simulink model "IndustrialMicrogrid"  (R2025a)
settings: Solver=FixedStepAuto  StartTime=0.0  StopTime=8  FixedStep=Ts  RelTol=1e-3
PostLoadFcn:
  | IndustrialMicrogridInputData
  | GfmGridFormingConverterInputParameters
model workspace (MAT data in the model file):
  caseNum = 2
undefined symbols (not defined in the file): base, BESS, DiscIntNeverNeededParam, grid, Grid, gridInverter, machine, microgrid, PV, PVInverter, PVTransformer, scrFactorRg, scrFactorXg, transformer, Transition_and_Dispatch_ControlModeType, Ts
libraries: ee_lib x126, fl_lib x91, eeGeneralControl x73, nesl_utility x50, nesl_utility_internal x46, simulink x30, eeTransforms x11, eeSinusoidalMeasurementV2 x5, eeTotalHarmonicDistorsion x4, slpidlib x3, simulink_extras x2, eePowerMeasurement x2
(part 5 of 12)

== system IndustrialMicrogrid/MG2 Processing, Lighting and Auxiliary Loads/Motor Loads ==
  Asynchronous Machine Squirrel Cage (fundamental) : ee_lib/Electromechanical/Asynchronous/Induction Machine Squirrel Cage  port_option=ee.enum.threePhasePort.composite  SRated=750000 V*A  VRated=4160 V  FRated=60 Hz  nPolePairs=2  param_unit=ee.enum.unit.si  squirrel_cage=ee.enum.squirrelcage.Single  zero_sequence=ee.enum.park.zerosequence.exclude  initialization_option=ee.enum.asm.initialization.fluxvariables  Rs=0.016744*7 Ohm  Xls=0.035490*7 Ohm  pu_Rs=0.0258  pu_Lls=0.0413  Rrd=0.009857*7 Ohm  Xlrd=0.04280*7 Ohm  pu_Rrd=0.0145  pu_Llrd=0.0424  Rrd1=0.28 Ohm  Xlrd1=0.82 Ohm  Rrd2=0.28 Ohm  Xlrd2=0.82 Ohm  pu_Rrd1=0.0290  pu_Llrd1=0.0848  pu_Rrd2=0.0290  pu_Llrd2=0.0848  Xm=111.90*7 Ohm  pu_Lm=1.7562  X0=0.4*7 Ohm  pu_L0=0.0413  saturation_option=ee.enum.saturation.exclude  saturation_i=[0, 4, 9, 18, 25, 34, 50, 68, 95, 120] A  saturation_v=[0, 88, 154, 198, 220, 242, 264, 286, 308, 327] V  pu_saturation_i=[0, .176, .396, .792, 1.1, 1.496, 2.2, 2.992, 4.18, 5.28]  pu_saturation_v=[0, .4, .7, .9, 1, 1.1, 1.2, 1.3, 1.4, 1.4864]  connection_option=ee.enum.Connection.delta1  angular_position_specify=off  angular_position_priority=None  angular_position=0 deg  angular_position_nominal_specify=off  angular_position_nominal_value=1  angular_position_nominal_unit=deg  pu_psids_specify=off  pu_psids_priority=None  pu_psids=0  pu_psids_nominal_specify=off  pu_psids_nominal_value=1  pu_psids_nominal_unit=1  pu_psiqs_specify=off  pu_psiqs_priority=None  pu_psiqs=0  pu_psiqs_nominal_specify=off  pu_psiqs_nominal_value=1  pu_psiqs_nominal_unit=1  pu_psi0s_specify=off  pu_psi0s_priority=None  pu_psi0s=0  pu_psi0s_nominal_specify=off  pu_psi0s_nominal_value=1  pu_psi0s_nominal_unit=1  pu_psidr_specify=off  pu_psidr_priority=None  pu_psidr=0  pu_psidr_nominal_specify=off  pu_psidr_nominal_value=1  pu_psidr_nominal_unit=1  pu_psiqr_specify=off  pu_psiqr_priority=None  pu_psiqr=0  pu_psiqr_nominal_specify=off  pu_psiqr_nominal_value=1  pu_psiqr_nominal_unit=1  pu_psidr1_specify=off  pu_psidr1_priority=None  pu_psidr1=0  pu_psidr1_nominal_specify=off  pu_psidr1_nominal_value=1  pu_psidr1_nominal_unit=1  pu_psiqr1_specify=off  pu_psiqr1_priority=None  pu_psiqr1=0  pu_psiqr1_nominal_specify=off  pu_psiqr1_nominal_value=1  pu_psiqr1_nominal_unit=1  pu_psidr2_specify=off  pu_psidr2_priority=None  pu_psidr2=0  pu_psidr2_nominal_specify=off  pu_psidr2_nominal_value=1  pu_psidr2_nominal_unit=1  pu_psiqr2_specify=off  pu_psiqr2_priority=None  pu_psiqr2=0  pu_psiqr2_nominal_specify=off  pu_psiqr2_nominal_value=1  pu_psiqr2_nominal_unit=1  psids_specify=off  psids_priority=None  psids=0 Wb  psids_nominal_specify=off  psids_nominal_value=1  psids_nominal_unit=Wb  psiqs_specify=off  psiqs_priority=None  psiqs=0 Wb  psiqs_nominal_specify=off  psiqs_nominal_value=1  psiqs_nominal_unit=Wb  psi0s_specify=off  psi0s_priority=None  psi0s=0 Wb  psi0s_nominal_specify=off  psi0s_nominal_value=1  psi0s_nominal_unit=Wb  psidr_specify=off  psidr_priority=None  psidr=0 Wb  psidr_nominal_specify=off  psidr_nominal_value=1  psidr_nominal_unit=Wb  psiqr_specify=off  psiqr_priority=None  psiqr=0 Wb  psiqr_nominal_specify=off  psiqr_nominal_value=1  psiqr_nominal_unit=Wb  psidr1_specify=off  psidr1_priority=None  psidr1=0 Wb  psidr1_nominal_specify=off  psidr1_nominal_value=1  psidr1_nominal_unit=Wb  psiqr1_specify=off  psiqr1_priority=None  psiqr1=0 Wb  psiqr1_nominal_specify=off  psiqr1_nominal_value=1  psiqr1_nominal_unit=Wb  psidr2_specify=off  psidr2_priority=None  psidr2=0 Wb  psidr2_nominal_specify=off  psidr2_nominal_value=1  psidr2_nominal_unit=Wb  psiqr2_specify=off  psiqr2_priority=None  psiqr2=0 Wb  psiqr2_nominal_specify=off  psiqr2_nominal_value=1  psiqr2_nominal_unit=Wb  slip_specify=on  slip_priority=None  slip=1  slip_nominal_specify=off  slip_nominal_value=1  slip_nominal_unit=1  real_power_generated_specify=on  real_power_generated_priority=None  real_power_generated=0 W  real_power_generated_nominal_specify=off  real_power_generated_nominal_value=1  real_power_generated_nominal_unit=W  mechanical_power_consumed_specify=on  mechanical_power_consumed_priority=None  mechanical_power_consumed=0 W  mechanical_power_consumed_nominal_specify=off  mechanical_power_consumed_nominal_value=1  mechanical_power_consumed_nominal_unit=W  Tmeas=298.15 K  alpha=3.93e-3 1/K  alpha_cage=4.4e-3 1/K  stator_thermal_mass=100 J/K  rotor_thermal_mass=200 J/K  temperatureA_specify=off  temperatureA_priority=High  temperatureA=25 degC  temperatureA_nominal_specify=off  temperatureA_nominal_value=1  temperatureA_nominal_unit=degC  temperatureB_specify=off  temperatureB_priority=High  temperatureB=25 degC  temperatureB_nominal_specify=off  temperatureB_nominal_value=1  temperatureB_nominal_unit=degC  temperatureC_specify=off  temperatureC_priority=High  temperatureC=25 degC  temperatureC_nominal_specify=off  temperatureC_nominal_value=1  temperatureC_nominal_unit=degC  temperatureR_specify=off  temperatureR_priority=High  temperatureR=25 degC  temperatureR_nominal_specify=off  temperatureR_nominal_value=1  temperatureR_nominal_unit=degC
      settings: InternalSimscapePortConfiguration="{\"Bottom\":[],\"Left\":[{\"id\":\"R\",\"label\":\"R\",\"type\":\"foundation.mechanical.rotational.rotational\"},{\"id\":\"C\",\"label\":\"C\",\"type\":\"foundation.mechanical.rotational.rotational\"}],\"Right\":[{\"id\":\"pu_output\",\"label\":\"pu\",\"type\":\"output\"},{\"id\":\"N1\",\"label\":\"~1\",\"type\":\"foundation.electrical.three_phase\"},{\"id\":\"N2\",\"label\":\"~2\",\"type\":\"foundation.electrical.three_phase\"}],\"Top\":[]}"
  Electrical Reference1 : fl_lib/Electrical/Electrical Elements/Electrical Reference
  Neutral Port (Three-Phase) : ee_lib/Connectors & References/Neutral Port (Three-Phase)  G_parasitic=1e-8 1/Ohm
      settings: InternalSimscapePortConfiguration="{\"Bottom\":[],\"Left\":[{\"id\":\"N\",\"label\":\"~\",\"type\":\"foundation.electrical.three_phase\"}],\"Right\":[{\"id\":\"n\",\"label\":\"n\",\"type\":\"foundation.electrical.electrical\"}],\"Top\":[]}"
  Subsystem : Subsystem
  ~ : PMIOPort  Side=Right
  connections:
  Subsystem/LConn2 -- Asynchronous Machine Squirrel Cage (fundamental)/LConn2
  Subsystem/LConn1 -- Asynchronous Machine Squirrel Cage (fundamental)/LConn1
  Neutral Port (Three-Phase)/RConn1 -- Electrical Reference1/LConn1
  Asynchronous Machine Squirrel Cage (fundamental)/RConn2 -- ~/RConn1
  Asynchronous Machine Squirrel Cage (fundamental)/RConn3 -- Neutral Port (Three-Phase)/LConn1

== system IndustrialMicrogrid/Operator Room/MG1 ==
  MG1 : Inport
  mLoad : Inport  Port=2
  mLoad3 : Inport  Port=3
  mTieine : Inport  Port=4
  "Measurements and Visualizations " : Subsystem
  Microgrid Control : Subsystem
  Monitoring of system performance : Subsystem
  Control Room MG1 : Outport
  Visualization MG1 : Outport  Port=2
  wires:
  MG1/1 -> Microgrid Control/1(MGController), "Measurements and Visualizations "/1(MG1)
  "Measurements and Visualizations "/1(Visualization) -> Monitoring of system performance/1(Visualization), Visualization MG1/1  "Visualization"
  Microgrid Control/1(CtrlRm) -> Control Room MG1/1
  mLoad/1 -> "Measurements and Visualizations "/2(mLoad)
  mTieine/1 -> "Measurements and Visualizations "/4(mTieline)
  mLoad3/1 -> "Measurements and Visualizations "/3(mLoad3)

== system IndustrialMicrogrid/Operator Room/MG2 ==
  MG2 : Inport
  mPV : Inport  Port=2
  mLoad2 : Inport  Port=3
  mPowerCentre : Inport  Port=4
  Measurements and Visualizations : Subsystem
  Microgrid Control : Subsystem
  Monitoring of system performance : Subsystem  SystemSampleTime=1e-3
  Visualization MG2 : Outport
  Control Room MG2 : Outport  Port=2
  wires:
  MG2/1 -> Microgrid Control/1(MGController), Measurements and Visualizations/1(MG2)
  Measurements and Visualizations/1(Visualization) -> Monitoring of system performance/1(Visualization), Visualization MG2/1
  mLoad2/1 -> Measurements and Visualizations/3(mLoad2)
  mPV/1 -> Measurements and Visualizations/2(mPV)
  Microgrid Control/1(CtrlRm) -> Control Room MG2/1
  mPowerCentre/1 -> Measurements and Visualizations/4(mPowerCentre)  "mPowerCentre"

== system IndustrialMicrogrid/Selected Results/MG1 ==
  BusElementIn : Inport  PortName=Visualization1  Element=MG1.Grid.activePower
  BusElementIn3 : Inport  PortName=Visualization1  Element=MG1.Grid.reactivePower
  BusElementIn1 : Inport  PortName=Visualization1  Element=MG1.BESS.activePower
  BusElementIn2 : Inport  PortName=Visualization1  Element=MG1.BESS.reactivePower
  BusElementIn4 : Inport  PortName=Visualization1  Element=MG1.Load.activePower
  BusElementIn5 : Inport  PortName=Visualization1  Element=MG1.Load.reactivePower
  Bus Creator2 : BusCreator  Inputs=3
  Bus Creator3 : BusCreator  Inputs=3
  MG1 : Scope  NumInputPorts=2
      settings: Title=Active Power (kW)  ActiveDisplayYMinimum=-0.09926  ActiveDisplayYMaximum=0.85966  DataLoggingDecimation=10
  wires:
  BusElementIn5/1 -> Bus Creator3/3  "Load Reactive Power"
  BusElementIn3/1 -> Bus Creator3/1  "Grid Reactive Power"
  Bus Creator3/1 -> MG1/2
  Bus Creator2/1 -> MG1/1
  BusElementIn4/1 -> Bus Creator2/3  "Load Active Power"
  BusElementIn/1 -> Bus Creator2/1  "Grid Active Power"
  BusElementIn1/1 -> Bus Creator2/2  "BESS Active Power"
  BusElementIn2/1 -> Bus Creator3/2  "BESS Reactive Power"

== system IndustrialMicrogrid/Selected Results/MG2 ==
  Bus Element In4 : Inport  PortName=Visualization  Element=MG2.Grid.activePower
  Bus Element In8 : Inport  PortName=Visualization  Element=MG2.Grid.reactivePower
  Bus Element In5 : Inport  PortName=Visualization  Element=MG2.BESS.activePower
  Bus Element In9 : Inport  PortName=Visualization  Element=MG2.BESS.reactivePower
  Bus Element In6 : Inport  PortName=Visualization  Element=MG2.Load.activePower
  Bus Element In10 : Inport  PortName=Visualization  Element=MG2.Load.reactivePower
  Bus Element In7 : Inport  PortName=Visualization  Element=MG2.PV.activePower
  Bus Element In1 : Inport  PortName=Visualization  Element=MG2.Diesel.activePower
  Bus Element In2 : Inport  PortName=Visualization  Element=MG2.Diesel.reactivePower
  Bus Creator : BusCreator  Inputs=5
  Bus Creator1 : BusCreator  Inputs=4
  MG2 : Scope  NumInputPorts=2
      settings: Title=Active Power (kW)  ActiveDisplayYMinimum=-0.99068  ActiveDisplayYMaximum=1.03601  DataLoggingDecimation=10  DataLoggingVariableName=ScopeData2
  wires:
  Bus Element In10/1 -> Bus Creator1/3  "Load Reactive Power"
  Bus Element In2/1 -> Bus Creator1/4  "Diesel Reactive Power"
  Bus Element In6/1 -> Bus Creator/3  "Load Active Power"
  Bus Element In1/1 -> Bus Creator/5  "Diesel Active Power"
  Bus Element In8/1 -> Bus Creator1/1  "Grid Reactive Power"
  Bus Element In4/1 -> Bus Creator/1  "Grid Active Power"
  Bus Creator/1 -> MG2/1
  Bus Creator1/1 -> MG2/2
  Bus Element In9/1 -> Bus Creator1/2  "BESS Reactive Power"
  Bus Element In7/1 -> Bus Creator/4  "PV Active Power"
  Bus Element In5/1 -> Bus Creator/2  "BESS Active Power"

== system IndustrialMicrogrid/MG1 Drilling Loads/Subsystem2/Subsystem ==
  Gain : Gain  Gain=60/(2*pi)
  Ideal Rotational Motion Sensor : fl_lib/Mechanical/Mechanical Sensors/Ideal Rotational Motion Sensor  reference=foundation.enum.MeasurementReference.difference  acceleration_port=false  velocity_port=true  position_port=false  wrap_angle=false  offset=0 rad
      settings: InternalSimscapePortConfiguration="{\"Bottom\":[],\"Left\":[{\"id\":\"R\",\"label\":\"R\",\"type\":\"foundation.mechanical.rotational.rotational\"}],\"Right\":[{\"id\":\"C\",\"label\":\"C\",\"type\":\"foundation.mechanical.rotational.rotational\"},{\"id\":\"W\",\"label\":\"W\",\"type\":\"output\"}],\"Top\":[]}"
  Machine Mechanical Power : ee_lib/Electromechanical/Mechanical/Machine Mechanical Power  power_sign=1  SRated=132000 A*V  FRated=60 Hz  nPolePairs=2  inputUnit=ee.enum.unit.si  torque_factor=2  inertia_option=2  J=10 kg*m^2  H=3.525 W*s/(A*V)  damper_option=2  D=39.0509 N*m*s/rad  pu_D=0.01  initialization_option=2  fMechanical0=60 Hz  fElectrical0=60 Hz
      settings: InternalSimscapePortConfiguration="{\"Bottom\":[],\"Left\":[{\"id\":\"Pm\",\"label\":\"Pm\",\"type\":\"input\"}],\"Right\":[{\"id\":\"R\",\"label\":\"R\",\"type\":\"foundation.mechanical.rotational.rotational\"},{\"id\":\"C\",\"label\":\"C\",\"type\":\"foundation.mechanical.rotational.rotational\"}],\"Top\":[]}"
  Mechanical Rotational Reference : fl_lib/Mechanical/Rotational Elements/Mechanical Rotational Reference
  PS-Simulink Converter : nesl_utility/PS-Simulink Converter  PhysicalDomain=network_engine_domain  SubClassName=ps_output  LeftPortType=input  RightPortType=output  PseudoPeriodic=off  Frequencies=[]  VectorFormat=inherit  Unit=inherit  AffineConversion=off
  Power : Constant  Value=120000
  Scope : Scope
      settings: ActiveDisplayYMinimum=-225.10191  ActiveDisplayYMaximum=2025.01132
  Simulink-PS Converter2 : nesl_utility/Simulink-PS Converter  PhysicalDomain=network_engine_domain  SubClassName=ps_input  LeftPortType=input  RightPortType=output  PseudoPeriodic=off  Frequencies=[]  NoiseDistribution=none  NoiseParameters=[]  Unit=1  AffineConversion=off  FilteringAndDerivatives=provide  SimscapeFilterOrder=1  InputFilterTimeConstant=0.001  UdotUserProvided=0
  Conn1 : PMIOPort  Side=Left
  Conn2 : PMIOPort  Port=2  Side=Left
  wires:
  PS-Simulink Converter/1 -> Gain/1
  Gain/1 -> Scope/1
  Power/1 -> Simulink-PS Converter2/1
  connections:
  PS-Simulink Converter/LConn1 -- Ideal Rotational Motion Sensor/RConn2
  Simulink-PS Converter2/RConn1 -- Machine Mechanical Power/LConn1
  Conn1/RConn1 -- Ideal Rotational Motion Sensor/LConn1 -- Machine Mechanical Power/RConn1
  Conn2/RConn1 -- Mechanical Rotational Reference/LConn1 -- Machine Mechanical Power/RConn2 -- Ideal Rotational Motion Sensor/RConn1

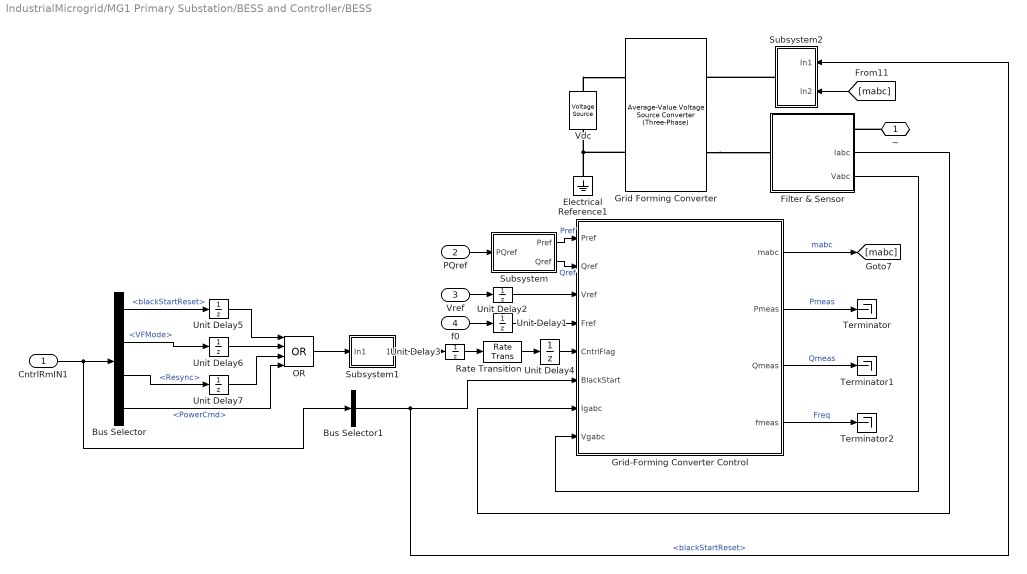
== system IndustrialMicrogrid/MG1 Primary Substation/BESS and Controller/BESS ==
  CntrlRmIN1 : Inport
  PQref : Inport  Port=2
  Vref : Inport  Port=3
  f0 : Inport  Port=4
  Bus Selector : BusSelector  OutputSignals=blackStartReset,VFMode,Resync,PowerCmd
  Bus Selector1 : BusSelector  OutputSignals=blackStartReset
  Electrical Reference1 : fl_lib/Electrical/Electrical Elements/Electrical Reference
  Filter & Sensor : Subsystem
      settings: PortSchema="{\"entries\":[{\"content\":{\"sides\":[{\"content\":{\"connectorIds\":[\"LConn1\"]},\"type\":\"ConnectorPlacement.EquallySpacedRectSide\",\"uuid\":\"5c627029-5c46-4463-a56d-3c0d548081be\"},{\"content\":{\"connectorIds\":[\"RConn1\",\"Out1\",\"Out2\"],\"side\":\"RIGHT\"},\"type\":\"ConnectorPlacement.EquallySpacedRectSide\",\"uuid\":\"d3de53bd-f6e0-45a5-afd4-617ea9ce7251\"},{\"content\":{\"side\":\"TOP\"},\"type\":\"ConnectorPlacement.EquallySpacedRectSide\",\"uuid\":\"c70d941f-8675-4ee6-83a0-a3fe29a369a2\"}]},\"type\":\"ConnectorPlacement.EquallySpacedConnector\",\"uuid\":\"0413e876-b9ec-4f56-9035-1758cb4de394\"}],\"packageUris\":[\"http://schema.mathworks.com/mf0/Connector/R2020b\"],\"version\":\"1.0\"}"
      mask Display: image('$imagefile'); % Use "Edit Image" on toolstrip to change.
  Grid Forming Converter : ee_lib/Semiconductors & Converters/Converters/Average-Value Voltage Source Converter (Three-Phase)  port_option=ee.enum.threePhasePort.composite  frequency_option=ee.enum.converters.frequency.variable  input_option=ee.enum.converters.inputOption.ModWave  FRated=50 Hz  losses_parameterization=ee.enum.converters.losses.fixed  Pfixed=1 W  ks=0.01  kc1=1.7 V  kc2=0.01 Ohm  Ploss_vect=[100, 800, 1870, 3250, 4900] W  Irms_vect=[10, 100, 200, 300, 400] A  Vdc_nom=300 V  thermal_mass=30000 J/K  temperature_specify=off  temperature_priority=High  temperature=298.15 K  temperature_nominal_specify=off  temperature_nominal_value=1  temperature_nominal_unit=K
      settings: InternalSimscapePortConfiguration="{\"Bottom\":[],\"Left\":[{\"id\":\"ModWave\",\"label\":\"ModWave\",\"type\":\"input\"},{\"id\":\"N\",\"label\":\"~\",\"type\":\"foundation.electrical.three_phase\"}],\"Right\":[{\"id\":\"p\",\"label\":\"+\",\"type\":\"foundation.electrical.electrical\"},{\"id\":\"n\",\"label\":\"-\",\"type\":\"foundation.electrical.electrical\"}],\"Top\":[]}"
  Grid-Forming Converter Control : Subsystem  mask(Grid Forming Controller){power=gridInverter.apparentPower*1e3, girdLineVoltage=gridInverter.lineRMSVoltage, powerFreq=gridInverter.frequency, dcBusVoltage=gridInverter.DCVoltage, measSampleTime=gridInverter.measurementSampleTime, powerControl=Virtual Synchronous Machine, activePowerSampleTime=gridInverter.droopControl.sampleTime, droopSlope=gridInverter.droopControl.freqSlopeMp, droopT1=gridInverter.droopControl.T1, droopT2=gridInverter.droopControl.T2, droopTC=gridInverter.droopControl.lpfTimeConst, vsmPmeasFilterTC=gridInverter.vsm.PmeasTimeConst, vsmFreqDroop=gridInverter.vsm.freqDroop, vsmInertiaTC=gridInverter.vsm.inertiaConstant, vsmDampingConst=gridInverter.vsm.dampingCoefficent/10, dampingPowerMaxLimit=gridInverter.vsm.maxDampingPower-0.2, dampingPowerMinLimit=gridInverter.vsm.minDampingPower, freqMeasTimeConst=gridInverter.freqMeasTimeConst, freqOption=Constant Frequency Reference, voltreference=gridInverter.Qcontrol.voltageReference, QVoltFilterTC=gridInverter.Qcontrol.QmeasTimeConst, QVoltDroop=gridInverter.Qcontrol.voltageDroop, currentLimit=Virtual Impedance, maxSatCurrentLimit=gridInverter.currentLimit.maxSaturationCurrent, maxVICurrentLimit=gridInverter.currentLimit.viCurrentLimit, ctLimitVirtualImp=gridInverter.currentLimit.virImpResistanceCoeff, ctLimitXbyR=gridInverter.currentLimit.virImpXbyR, ctLimitDelayTime=gridInverter.currentLimit.maxSaturationDelay, currentSatTime=gridInverter.currentLimit.satCurrentRunTime, currentVITimeConst=gridInverter.currentLimit.viFilterTimeConst, voltControlTs=gridInverter.controller.VoltageControlSampleTime, vdPGain=gridInverter.controller.voltControllerKp, VdIGain=gridInverter.controller.voltControllerKi, VdMaxCt=gridInverter.controller.voltageMaxId, VdMinCt=gridInverter.controller.voltageMinId, VqPGain=gridInverter.controller.voltControllerKp, VqIGain=gridInverter.controller.voltControllerKi, VqMaxCt=gridInverter.controller.voltageMaxIq, VqMinCt=gridInverter.controller.voltageMinIq, vdvqLPFTimeConst=gridInverter.controller.voltMeasTimeConst, currentControlTs=gridInverter.controller.CurrentControlSampleTime, filterInductance=gridInverter.L, IdPGain=gridInverter.controller.ctControllerKp, IdIGain=gridInverter.controller.ctControllerKi, IqPGain=gridInverter.controller.ctControllerKp, IqIGain=gridInverter.controller.ctControllerKi}
      mask prompts: power "Grid forming converter power (VA)"; girdLineVoltage "Grid line voltage (V)"; powerFreq "Grid frequency (Hz)"; dcBusVoltage "DC bus voltage"; measSampleTime "Measurement sample time"; powerControl "Active Power Control"; activePowerSampleTime "Sample time (s)"; droopSlope "Power droop slope (pu, Hz/W)"; droopT1 "Lead-Lag numerator time constant (s)"; droopT2 "Lead-Lag denominator time constant (s)"; droopTC "Filter cut-off time constant (s)"; vsmPmeasFilterTC "Power measurement filter time constant (s)"; vsmFreqDroop "Frequency droop (pu,  W/Hz)"; vsmInertiaTC "Inertia constant M (pu)"; vsmDampingConst "Damping constant (pu/Hz)"; dampingPowerMaxLimit "Damping power maximum limit (pu)"; dampingPowerMinLimit "Damping power minimum limit (pu)"; freqMeasTimeConst "Frequency measurement time constant (s)"; freqOption "Damping power fequency option"; voltreference "Voltage reference value (pu)"; QVoltFilterTC "Power measurement filter time constant (s)"; QVoltDroop "Voltage droop (pu, V/VAR)"; currentLimit "Current limiting method"; maxSatCurrentLimit "Maximum current saturation (pu)"; maxVICurrentLimit "Maximum virtual impedance current (pu)"; ctLimitVirtualImp "Virtual impedance coefficient (pu.Ohm/pu.A)"; ctLimitXbyR "Virtual X/R ratio"; ctLimitDelayTime "Maximum current delay time (s)"; currentSatTime "Current limiting run time (s)"; currentVITimeConst "Filter time constant (s)"; voltControlTs "Controller sample time (s)"; vdPGain "Vd proportional gain"; VdIGain "Vd integral gain"; VdMaxCt "Vd maximum current limit (A)"; VdMinCt "Vd minimum current limit (A)"; VqPGain "Vq proportional gain"; VqIGain "Vq integral gain"; VqMaxCt "Vq maximum current limit (A)"; VqMinCt "Vq minimum current limit (A)"; vdvqLPFTimeConst "Voltage measurement filter time constant (s)"; currentControlTs "Controller sample time (s)"; filterInductance "Filter inductance (H)"; IdPGain "Id proportional gain"; IdIGain "Id integral gain"; IqPGain "Iq proportional gain"; IqIGain "Iq integral gain"
      mask help: This block implements the grid forming controller with fault ride through capability. Input to the controller are active and reactive power reference in per unit and the sensed three-phase phase current in amphere and phase voltage in volts.
      mask init:
      | powerChoice = get_param(gcb,'powerControl');
      | currentChoice = get_param(gcb,'currentLimit');
      | 
      | powerloc = [gcb, '/Power Control/ActivePowerControl']; 
      | currentloc = [gcb, '/Current Limiting/CurrentLimitingMethod'];
      | freqLoc = [gcb,'/Power Control/ActivePowerControl/vsmControl/Damping Frequency'];
      | 
      | switch powerChoice
      |     case 'Virtual Synchronous Machine'
      |         set_param(powerloc, 'LabelModeActiveChoice', 'vsm');
      |         dampingFreqChoice = get_param(gcb,'freqOption');
      |         if strcmp(dampingFreqChoice,'Use Grid Frequency Measurement')
      |             set_param(freqLoc, 'LabelModeActiveChoice', 'freqMeas');
      |         else
      |             set_param(freqLoc, 'LabelModeActiveChoice', 'constFreq');
      |         end
      |     case 'Droop Control'
      |          set_param(powerloc, 'LabelModeActiveChoice', 'droop');
      |    otherwise
      |         disp('Choose proper active power control method')
      | end
      | switch currentChoice
      |     case 'Virtual Impedance'
      |           set_param(currentloc, 'LabelModeActiveChoice', 'virimp');
      |     case 'Current Limiting'
      |          set_param(currentloc, 'LabelModeActiveChoice', 'ctSat');
      |     case 'Combining Virtual Impedance and Current Limiting'
      |             set_param(currentloc, 'LabelModeActiveChoice', 'both');
      |     otherwise
      |         disp('Choose proper current limiting method')
      | end
      mask TypeOptions powerControl: Virtual Synchronous Machine | Droop Control
      mask Callback powerControl:
      | h = Simulink.Mask.get(gcb);
      | slectedActivePowerControl=get_param(gcb,'powerControl');
      | %slectedActivePowerControl = h.Parameters(find(string({h.Parameters.Name}) == 'powerControl')).Value;
      | switch slectedActivePowerControl
      |     case 'Virtual Synchronous Machine'
      |         h.Parameters(find(string({h.Parameters.Name}) == 'droopSlope')).Visible = 'off';
      |         h.Parameters(find(string({h.Parameters.Name}) == 'droopTC')).Visible = 'off';
      |         h.Parameters(find(string({h.Parameters.Name}) == 'droopT1')).Visible = 'off';
      |         h.Parameters(find(string({h.Parameters.Name}) == 'droopT2')).Visible = 'off';
      |         h.Parameters(find(string({h.Parameters.Name}) == 'vsmPmeasFilterTC')).Visible = 'on';
      |         h.Parameters(find(string({h.Parameters.Name}) == 'vsmFreqDroop')).Visible = 'on';
      |         h.Parameters(find(string({h.Parameters.Name}) == 'vsmInertiaTC')).Visible = 'on';
      |         h.Parameters(find(string({h.Parameters.Name}) == 'vsmDampingConst')).Visible = 'on';
      |         h.Parameters(find(string({h.Parameters.Name}) == 'dampingPowerMaxLimit')).Visible = 'on';
      |         h.Parameters(find(string({h.Parameters.Name}) == 'dampingPowerMinLimit')).Visible = 'on';
      |         h.Parameters(find(string({h.Parameters.Name}) == 'freqOption')).Visible = 'on';
      |         h.Parameters(find(string({h.Parameters.Name}) == 'freqMeasTimeConst')).Visible = 'on';
      |     case 'Droop Control'
      |         h.Parameters(find(string({h.Parameters.Name}) == 'droopSlope')).Visible = 'on';
      |         h.Parameters(find(string({h.Parameters.Name}) == 'droopTC')).Visible = 'on';
      |         h.Parameters(find(string({h.Parameters.Name}) == 'droopT1')).Visible = 'on';
      |         h.Parameters(find(string({h.Parameters.Name}) == 'droopT2')).Visible = 'on';
      |         h.Parameters(find(string({h.Parameters.Name}) == 'vsmPmeasFilterTC')).Visible = 'off';
      |         h.Parameters(find(string({h.Parameters.Name}) == 'vsmFreqDroop')).Visible = 'off';
      |         h.Parameters(find(string({h.Parameters.Name}) == 'vsmInertiaTC')).Visible = 'off';
      |         h.Parameters(find(string({h.Parameters.Name}) == 'vsmDampingConst')).Visible = 'off';
      |         h.Parameters(find(string({h.Parameters.Name}) == 'dampingPowerMaxLimit')).Visible = 'off';
      |         h.Parameters(find(string({h.Parameters.Name}) == 'dampingPowerMinLimit')).Visible = 'off';
      |         h.Parameters(find(string({h.Parameters.Name}) == 'freqOption')).Visible = 'off';
      |         h.Parameters(find(string({h.Parameters.Name}) == 'freqMeasTimeConst')).Visible = 'on';
      | 
      |     otherwise
      |         disp('Choose proper active power control method')
      | end
      mask TypeOptions freqOption: Use Grid Frequency Measurement | Constant Frequency Reference
      mask TypeOptions currentLimit: Virtual Impedance | Current Limiting | Combining Virtual Impedance and Current Limiting
      mask Callback currentLimit:
      | currentLimit = 1;
      | h = Simulink.Mask.get(gcb);
      | currentLimitControl=get_param(gcb,'currentLimit');
      | %slectedActivePowerControl = h.Parameters(find(string({h.Parameters.Name}) == 'powerControl')).Value;
      | switch currentLimitControl
      |     case 'Virtual Impedance'
      |         h.Parameters(find(string({h.Parameters.Name}) == 'maxVICurrentLimit')).Visible = 'on';
      |         h.Parameters(find(string({h.Parameters.Name}) == 'ctLimitVirtualImp')).Visible = 'on';
      |         h.Parameters(find(string({h.Parameters.Name}) == 'ctLimitXbyR')).Visible = 'on';
      |         h.Parameters(find(string({h.Parameters.Name}) == 'maxSatCurrentLimit')).Visible = 'off';
      |         h.Parameters(find(string({h.Parameters.Name}) == 'ctLimitDelayTime')).Visible = 'off';
      |         h.Parameters(find(string({h.Parameters.Name}) == 'currentSatTime')).Visible = 'off';
      |         h.Parameters(find(string({h.Parameters.Name}) == 'currentVITimeConst')).Visible = 'on';
      | 
      | 
      |     case 'Current Limiting'
      |         h.Parameters(find(string({h.Parameters.Name}) == 'maxVICurrentLimit')).Visible = 'off';
      |         h.Parameters(find(string({h.Parameters.Name}) == 'ctLimitVirtualImp')).Visible = 'off';
      |         h.Parameters(find(string({h.Parameters.Name}) == 'ctLimitXbyR')).Visible = 'off';
      |         h.Parameters(find(string({h.Parameters.Name}) == 'maxSatCurrentLimit')).Visible = 'on';
      |         h.Parameters(find(string({h.Parameters.Name}) == 'ctLimitDelayTime')).Visible = 'on';
      |         h.Parameters(find(string({h.Parameters.Name}) == 'currentSatTime')).Visible = 'off';
      |         h.Parameters(find(string({h.Parameters.Name}) == 'currentVITimeConst')).Visible = 'off';
      | 
      |     case 'Combining Virtual Impedance and Current Limiting'
      |         h.Parameters(find(string({h.Parameters.Name}) == 'maxVICurrentLimit')).Visible = 'on';
      |         h.Parameters(find(string({h.Parameters.Name}) == 'ctLimitVirtualImp')).Visible = 'on';
      |         h.Parameters(find(string({h.Parameters.Name}) == 'ctLimitXbyR')).Visible = 'on';
      |         h.Parameters(find(string({h.Parameters.Name}) == 'maxSatCurrentLimit')).Visible = 'on';
      |         h.Parameters(find(string({h.Parameters.Name}) == 'ctLimitDelayTime')).Visible = 'off';
      |         h.Parameters(find(string({h.Parameters.Name}) == 'currentSatTime')).Visible = 'on';
      |         h.Parameters(find(string({h.Parameters.Name}) == 'currentVITimeConst')).Visible = 'on';
      | 
      |     otherwise
      |         disp('Choose proper current limiting method')
      | end
      mask DialogControl ParameterGroupVar Prompt: Grid Forming Control Parameters
      mask DialogControl Container8 Prompt: Grid-forming Converter Specification
      mask DialogControl Pcontrolgrp Prompt: Active Power Controller Parameters
      mask DialogControl QcontrolGrp Prompt: Reactive Power Controller Parameters
      mask DialogControl faultRideThroughGrp Prompt: Fault Ride Through Parameters
      mask DialogControl voltControlgrp Prompt: Voltage Controller Parameters
      mask DialogControl Container15currentContGrp Prompt: Current Controller Parameters
      mask Display: image('$imagefile'); % Use "Edit Image" on toolstrip to change.
  OR : Logic  Operator=OR  Inputs=4  IconShape=distinctive  AllPortsSameDT=off  OutDataTypeStr=boolean
  Rate Transition : RateTransition
  Subsystem : Subsystem
  Subsystem1 : Subsystem
  Subsystem2 : Subsystem
  Terminator : Terminator
  Terminator1 : Terminator
  Terminator2 : Terminator
  Unit Delay{1..4} (4 alike) : UnitDelay  InitialCondition=1  SampleTime=Ts  HasFrameUpgradeWarning=on
  Unit Delay5 : UnitDelay  SampleTime=Ts  HasFrameUpgradeWarning=on
  Unit Delay6 : UnitDelay  SampleTime=Ts  HasFrameUpgradeWarning=on
  Unit Delay7 : UnitDelay  SampleTime=Ts  HasFrameUpgradeWarning=on
  Vdc : ee_lib/Sources/Voltage Source  dc_voltage=gridInverter.DCVoltage V  ac_voltage=0 V  ac_shift=0 rad  ac_frequency=0 Hz  noise_mode=ee.enum.sources.noise.Disabled  PSD=0 V^2/Hz  sample_time=1e-3 s  repeatability=ee.enum.sources.repeatability.NotRepeatable  user_seed=0  auto_seed=545404223  i_specify=off  i_priority=None  i=0 A  i_nominal_specify=off  i_nominal_value=1  i_nominal_unit=A  v_specify=off  v_priority=None  v=0 V  v_nominal_specify=off  v_nominal_value=1  v_nominal_unit=V
  "~ " : PMIOPort  Side=Left
  wires:
  Grid-Forming Converter Control/3(Qmeas) -> Terminator1/1  "Qmeas"
  Grid-Forming Converter Control/2(Pmeas) -> Terminator/1  "Pmeas"
  Subsystem/1(Pref) -> Grid-Forming Converter Control/1(Pref)  "Pref"
  Grid-Forming Converter Control/1(mabc) -> [mabc]  "mabc"
  Subsystem/2(Qref) -> Grid-Forming Converter Control/2(Qref)  "Qref"
  Grid-Forming Converter Control/4(fmeas) -> Terminator2/1  "Freq"
  CntrlRmIN1/1 -> Bus Selector1/1, Bus Selector/1
  PQref/1 -> Subsystem/1(PQref)
  Vref/1 -> Unit Delay2/1
  f0/1 -> Unit Delay1/1
  Subsystem1/1(Out1) -> Unit Delay3/1
  Rate Transition/1 -> Unit Delay4/1
  Unit Delay4/1 -> Grid-Forming Converter Control/5(CntrlFlag)
  Unit Delay3/1 -> Rate Transition/1
  Unit Delay1/1 -> Grid-Forming Converter Control/4(Fref)
  Unit Delay2/1 -> Grid-Forming Converter Control/3(Vref)
  Unit Delay7/1 -> OR/3
  Unit Delay6/1 -> OR/2
  Unit Delay5/1 -> OR/1
  OR/1 -> Subsystem1/1(In1)
  [mabc] -> Subsystem2/2(In2)
  Filter & Sensor/1(Iabc) -> Grid-Forming Converter Control/7(Igabc)
  Filter & Sensor/2(Vabc) -> Grid-Forming Converter Control/8(Vgabc)
  Bus Selector/3 -> Unit Delay7/1  "<Resync>"
  Bus Selector/2 -> Unit Delay6/1  "<VFMode>"
  Bus Selector/1 -> Unit Delay5/1  "<blackStartReset>"
  Bus Selector/4 -> OR/4  "<PowerCmd>"
  Bus Selector1/1 -> Subsystem2/1(In1), Grid-Forming Converter Control/6(BlackStart)  "<blackStartReset>"
  connections:
  Electrical Reference1/LConn1 -- Grid Forming Converter/RConn2 -- Vdc/RConn1
  "~ "/RConn1 -- Filter & Sensor/RConn1
  Grid Forming Converter/LConn2 -- Filter & Sensor/LConn1
  Vdc/LConn1 -- Grid Forming Converter/RConn1
  Subsystem2/RConn1 -- Grid Forming Converter/LConn1

== system IndustrialMicrogrid/MG1 Primary Substation/BESS and Controller/BESS Converter Measurement  ==
  Current and Voltage Sensor (Three-Phase) : ee_lib/Sensors & Transducers/Current and Voltage Sensor (Three-Phase)  vMeasurementType=ee.enum.vmeasurement.lg  outputUnit=ee.enum.unit.pu  SRated=1e6 A*V  VRated=microgrid.voltage V  I_specify=off  I_priority=None  I=[ 0 0 0 ] A  I_nominal_specify=off  I_nominal_value=1  I_nominal_unit=A  V_specify=off  V_priority=None  V=[ 0 0 0 ] V  V_nominal_specify=off  V_nominal_value=1  V_nominal_unit=V
      settings: InternalSimscapePortConfiguration="{\"Bottom\":[],\"Left\":[{\"id\":\"N1\",\"label\":\"~1\",\"type\":\"foundation.electrical.three_phase\"}],\"Right\":[{\"id\":\"V_output\",\"label\":\"V\",\"type\":\"output\"},{\"id\":\"I_output\",\"label\":\"I\",\"type\":\"output\"},{\"id\":\"N2\",\"label\":\"~2\",\"type\":\"foundation.electrical.three_phase\"}],\"Top\":[]}"
  Low-Pass Filter (Discrete or Continuous) : eeGeneralControl/Low-Pass Filter (Discrete or Continuous)  K=1  T=0.02  B=inf  A=-inf  init_option=Inherited from block input  x0=0  Ts=Ts
  Low-Pass Filter (Discrete or Continuous)1 : eeGeneralControl/Low-Pass Filter (Discrete or Continuous)  K=1  T=0.02  B=inf  A=-inf  init_option=Inherited from block input  x0=0  Ts=Ts
  PS-Simulink Converter2 : nesl_utility_internal/PS-Simulink Converter  PhysicalDomain=network_engine_domain  SubClassName=ps_output  LeftPortType=input  RightPortType=output  PseudoPeriodic=off  Frequencies=[]  VectorFormat=1-D array  Unit=V  AffineConversion=off
  PS-Simulink Converter3 : nesl_utility_internal/PS-Simulink Converter  PhysicalDomain=network_engine_domain  SubClassName=ps_output  LeftPortType=input  RightPortType=output  PseudoPeriodic=off  Frequencies=[]  VectorFormat=1-D array  Unit=A  AffineConversion=off
  PS-Simulink Converter6 : nesl_utility_internal/PS-Simulink Converter  PhysicalDomain=network_engine_domain  SubClassName=ps_output  LeftPortType=input  RightPortType=output  PseudoPeriodic=off  Frequencies=[]  VectorFormat=1-D array  Unit=MW  AffineConversion=off
  PS-Simulink Converter7 : nesl_utility_internal/PS-Simulink Converter  PhysicalDomain=network_engine_domain  SubClassName=ps_output  LeftPortType=input  RightPortType=output  PseudoPeriodic=off  Frequencies=[]  VectorFormat=1-D array  Unit=MV*A  AffineConversion=off
  Power Sensor (Three-Phase)1 : ee_lib/Sensors & Transducers/Power Sensor (Three-Phase)  load_type=ee.enum.passive.type_balanced.balanced  f0=60 Hz  config=ee.enum.with_neutral.no  rho=1
      settings: InternalSimscapePortConfiguration="{\"Bottom\":[],\"Left\":[{\"id\":\"N1\",\"label\":\"~1\",\"type\":\"foundation.electrical.three_phase\"}],\"Right\":[{\"id\":\"N2\",\"label\":\"~2\",\"type\":\"foundation.electrical.three_phase\"}],\"Top\":[{\"id\":\"Pm\",\"label\":\"P\",\"type\":\"output\"},{\"id\":\"Qm\",\"label\":\"Q\",\"type\":\"output\"}]}"
  a1 : PMIOPort  Side=Left
  ~ : PMIOPort  Port=2  Side=Right
  Out Bus Element : Outport  PortName=mBESS1  Element=voltage
  Out Bus Element1 : Outport  PortName=mBESS1  Element=current
  Out Bus Element2 : Outport  PortName=mBESS1  Element=active power
  Out Bus Element3 : Outport  PortName=mBESS1  Element=reactive power
  wires:
  Low-Pass Filter (Discrete or Continuous)1/1 -> Out Bus Element2/1
  Low-Pass Filter (Discrete or Continuous)/1 -> Out Bus Element3/1
  PS-Simulink Converter3/1 -> Out Bus Element1/1
  PS-Simulink Converter7/1 -> Low-Pass Filter (Discrete or Continuous)/1
  PS-Simulink Converter6/1 -> Low-Pass Filter (Discrete or Continuous)1/1
  PS-Simulink Converter2/1 -> Out Bus Element/1
  connections:
  ~/RConn1 -- Power Sensor (Three-Phase)1/RConn1
  Power Sensor (Three-Phase)1/LConn3 -- PS-Simulink Converter7/LConn1
  Power Sensor (Three-Phase)1/LConn2 -- PS-Simulink Converter6/LConn1
  Current and Voltage Sensor (Three-Phase)/RConn2 -- PS-Simulink Converter3/LConn1
  PS-Simulink Converter2/LConn1 -- Current and Voltage Sensor (Three-Phase)/RConn1
  Current and Voltage Sensor (Three-Phase)/LConn1 -- a1/RConn1
  Power Sensor (Three-Phase)1/LConn1 -- Current and Voltage Sensor (Three-Phase)/RConn3

== system IndustrialMicrogrid/MG1 Primary Substation/BESS and Controller/BESS output filter and transformer1 ==
  10 kvar : ee_lib/Passive/RLC Assemblies/Wye-Connected Load  port_option=ee.enum.threePhasePort.composite  parameterization=ee.enum.rlc.parameterization.ratedpower  component_structure=ee.enum.rlc.structure.C  component_structure_PQ=ee.enum.rlc.structure.C  R=1 Ohm  L=0.001 H  C=1e-6 F  VRated=microgrid.voltage V  FRated=grid.frequency Hz  P=0 W  Qpos=0 A*V  Qneg=BESS.qBESSFilter A*V  R_parasitic=1e-6 Ohm  G_parasitic=1e-6 1/Ohm  R_parasitic_PQ=1e-6 Ohm  G_parasitic_PQ=1e-6 1/Ohm  Vmag0=microgrid.voltage V  Vang0=0 deg  Freq0=grid.frequency Hz  IL_specify=on  IL_priority=High  IL=[ 0 0 0 ] A  IL_nominal_specify=off  IL_nominal_value=1  IL_nominal_unit=A  VC_specify=on  VC_priority=High  VC=[ 0 0 0 ] V  VC_nominal_specify=off  VC_nominal_value=1  VC_nominal_unit=V
  Electrical Reference1 : fl_lib/Electrical/Electrical Elements/Electrical Reference
  Transformer 1 kV/13.8 kV : Subsystem
      mask Display: image('$imagefile'); % Use "Edit Image" on toolstrip to change.
  "~ " : PMIOPort  Side=Right
  ~ : PMIOPort  Port=2  Side=Left
  connections:
  Electrical Reference1/LConn1 -- 10 kvar/RConn1
  10 kvar/LConn1 -- Transformer 1 kV/13.8 kV/RConn1 -- "~ "/RConn1
  Transformer 1 kV/13.8 kV/LConn1 -- ~/RConn1

== system IndustrialMicrogrid/MG1 Primary Substation/Microgrid Controller/Breaker Control ==
  Bus Element In : Inport  PortName=BrKControl  Element=PCC
  CtrlRm BRK : Inport  Port=2
  Cast To Double1 : DataTypeConversion  OutDataTypeStr=double  SaturateOnIntegerOverflow=off  RndMeth=Floor
  Delay : Delay  DelayLength=1  InitialCondition=microgrid.PCC1BrkInitStatus
  Switch : Switch  Criteria=u2 > Threshold  SaturateOnIntegerOverflow=off  InputSameDT=off
  BrK Ctrl : Outport
  wires:
  Delay/1 -> Cast To Double1/1
  Bus Element In/1 -> Delay/1
  CtrlRm BRK/1 -> Switch/1, Switch/2
  Cast To Double1/1 -> Switch/3  "BRK Status"
  Switch/1 -> BrK Ctrl/1  "BRK Status"

== system IndustrialMicrogrid/MG1 Primary Substation/Microgrid Controller/Microgrid Control Functions ==
  PLL : Inport
  BESS Reactive Power : Inport  Port=2
  PCC Active Power : Inport  Port=3
  PCC Reactive Power : Inport  Port=4
  Bus Element In1 : Inport  Port=5  PortName=Status  Element=plannedIslandingEnable
  Bus Element In2 : Inport  Port=5  PortName=Status  Element=blackStartEnable
  Bus Element In4 : Inport  Port=5  PortName=Status  Element=resyncEnable
  Bus Element In3 : Inport  Port=5  PortName=Status  Element=resync
  Data Type Conversion : DataTypeConversion  OutDataTypeStr=boolean  SaturateOnIntegerOverflow=off  RndMeth=Floor
  Latency_Blackstart : Delay  DelayLength=1  SampleTime=Ts
  Latency_PlannedIsland : Delay  DelayLength=1  SampleTime=Ts
  Latency_Resync : Delay  DelayLength=1  SampleTime=Ts
  Model : ModelReference  ModelNameDialog=Resynchronization.slx  UsingDefaultArgumentValue=0,0,0,0,0,0,0,0,0,0,0  SimulationMode=Normal  ModelReferenceVersion=5.0  GridFrequency=gridFrequency  KpVolResynch=kpVoltage  KiVolResynch=kiVoltage  VoltageThreshold=voltageThreshold  kDroop=voltageDroop  KpFreResynch=kpFrequency  KiFreResynch=kiFrequency  FrequencyThreshold=frequencyThreshold  KpAngResynch=kpAngle  KiAngResynch=kiAngle  AngleThreshold=angleThreshold
  Model1 : ModelReference  ModelNameDialog=PlannedIsland.slx  UsingDefaultArgumentValue=0,0,0,0,0,0  SimulationMode=Normal  ModelReferenceVersion=5.0  KpPPlannedIsland=kpActive  KiPPlannedIsland=kiActive  ZeroActivePowerThreshold=activeThreshold  KpQPlannedIsland=kpReactive  KiQPlannedIsland=kiReactive  ZeroReactivePowerThreshold=reactiveThreshold
  Model2 : ModelReference  ModelNameDialog=Black_Start.slx  UsingDefaultArgumentValue=0,0,0,0,0,0,0,0  SimulationMode=Normal  ModelReferenceVersion=5.0  referenceFrequency=blackStartFrequency  controllerBlackStart=blackStartTime  voltageLevel1=level1  voltageLevel2=level2  voltageLevel3=level3  delayLevel1=delay1  delayLevel2=delay2  delayLevel3=delay3
      settings: PortSchema="{\"entries\":[{\"content\":{\"sides\":[{\"content\":{\"connectorIds\":[\"In1\",\"In2\"]},\"type\":\"ConnectorPlacement.EquallySpacedRectSide\",\"uuid\":\"43ba8e4b-663e-4345-aeb4-26821aebb17e\"},{\"content\":{\"connectorIds\":[\"Out2\",\"Out1\"],\"side\":\"RIGHT\"},\"type\":\"ConnectorPlacement.EquallySpacedRectSide\",\"uuid\":\"a8a82b84-e866-44f5-9bce-204b1ef747e6\"},{\"content\":{\"side\":\"TOP\"},\"type\":\"ConnectorPlacement.EquallySpacedRectSide\",\"uuid\":\"05fd1043-1a12-402f-89e0-8461a16f1a17\"}]},\"type\":\"ConnectorPlacement.EquallySpacedConnector\",\"uuid\":\"6310347e-2957-46fe-a759-6964c7aa5534\"}],\"packageUris\":[\"http://schema.mathworks.com/mf0/Connector/R2020b\"],\"version\":\"1.0\"}"
  Resync : Outport
  PlannedIslanding : Outport  Port=2
  BlackStart : Outport  Port=3
  Resync Status : Outport  Port=4
  PlannedIsland Status : Outport  Port=5
  BlackStart Status : Outport  Port=6
  wires:
  Model1/2 -> PlannedIslanding/1  "PlannedIslanding"
  PCC Reactive Power/1 -> Model1/3
  PCC Active Power/1 -> Model1/2
  Model/1 -> Latency_Resync/1
  Model1/1 -> Latency_PlannedIsland/1
  Bus Element In2/1 -> Model2/1
  Model2/1 -> BlackStart/1  "BlackStart"
  Bus Element In1/1 -> Model1/1
  Model/2 -> Resync/1  "Resync"
  Bus Element In3/1 -> Data Type Conversion/1
  Bus Element In4/1 -> Model/1
  BESS Reactive Power/1 -> Model/2
  PLL/1 -> Model2/2, Model/3
  Data Type Conversion/1 -> Model/4
  Latency_Resync/1 -> Resync Status/1
  Latency_PlannedIsland/1 -> PlannedIsland Status/1
  Model2/2 -> Latency_Blackstart/1
  Latency_Blackstart/1 -> BlackStart Status/1

== system IndustrialMicrogrid/MG1 Primary Substation/Microgrid Controller/Microgrid Supervisory Control ==
  Resync Status : Inport
  PlannedIslanding Status : Inport  Port=2
  BlackStart Status : Inport  Port=3
  Resync Enable : Inport  Port=4
  PlannedIslandEnable : Inport  Port=5
  UnplannedIslandingEnable : Inport  Port=6
  BlackStart Enable : Inport  Port=7
  Bus Element In : Inport  Port=8  PortName=mPLL  Element=Island.voltage
  Bus Element In1 : Inport  Port=8  PortName=mPLL  Element=Island.frequency
  Blackout Status1 : Inport  Port=9
  BreakerStatus : Inport  Port=10
  Bus Assignment : BusAssignment  AssignedSignals=mode
  Bus Creator : BusCreator  Inputs=3
  Bus Creator1 : BusCreator  Inputs=2
  Bus Creator2 : BusCreator  Inputs=3
  Bus Creator3 : BusCreator  Inputs=3
  Constant : Constant  Value=resyncDelay
  Constant1 : Constant  Value=plannedIslandingDelay
  Delay : Delay  DelayLength=1  InitialCondition=microgrid.PCC1BrkInitStatus  SampleTime=Ts
  Transition and Dispatch Control : Stateflow chart  TreatAsAtomicUnit=on  mask(Microgrid Transition and Dispatch Control){upperVoltageLimit=upperVoltagelimit, lowerVoltageLimit=lowerVoltageLimit, upperFrequencyLimit=upperFrequencyLimit, lowerFrequencyLimit=lowerFrequencyLimit}
      mask prompts: upperVoltageLimit "Max Voltage in pu"; lowerVoltageLimit "Min Voltage in pu"; upperFrequencyLimit "Max Frequency in Hz"; lowerFrequencyLimit "Min Frequency in Hz"
      mask help: This subsystem implements the transitions and the corresponding dispatch functions in the microgrid
  BrKControl : Outport
  Status : Outport  Port=2
  wires:
  PlannedIslanding Status/1 -> Bus Creator2/2  "status"
  PlannedIslandEnable/1 -> Bus Creator2/1  "enable"
  UnplannedIslandingEnable/1 -> Transition and Dispatch Control/2(UnplannedIslandingEnable)
  Bus Creator1/1 -> Transition and Dispatch Control/3(Island)  "Island"
  Bus Element In1/1 -> Bus Creator1/2  "frequency"
  Bus Element In/1 -> Bus Creator1/1  "voltage"
  Bus Creator/1 -> Transition and Dispatch Control/1(Resync)  "Resync"
  Constant/1 -> Bus Creator/3  "delay"
  Resync Status/1 -> Bus Creator/2  "status"
  Resync Enable/1 -> Bus Creator/1  "enable"
  Transition and Dispatch Control/1(BrKControl) -> BrKControl/1  "BrKControl"
  BreakerStatus/1 -> Delay/1
  Transition and Dispatch Control/2(Status) -> Bus Assignment/1
  Transition and Dispatch Control/3(Transition_and_Dispatch_ControlMode) -> Bus Assignment/2
  Bus Assignment/1 -> Status/1  "Status"
  Delay/1 -> Transition and Dispatch Control/4(BreakerStatus)
  Constant1/1 -> Bus Creator2/3  "delay"
  BlackStart Status/1 -> Bus Creator3/2  "status"
  Blackout Status1/1 -> Bus Creator3/3  "blackout"
  BlackStart Enable/1 -> Bus Creator3/1  "enable"
  Bus Creator3/1 -> Transition and Dispatch Control/6(BlackStart)  "BlackStart"
  Bus Creator2/1 -> Transition and Dispatch Control/5(PlannedIslanding)  "PlannedIslanding"

== system IndustrialMicrogrid/MG1 Primary Substation/PCC Measurements and PCC Breaker/Circuit Breaker ==
  BRK : Inport
  Data Type Conversion : DataTypeConversion  OutDataTypeStr=double  SaturateOnIntegerOverflow=off  RndMeth=Floor
  Open Resistance : Gain  Gain=1e5
  Phase Splitter : ee_lib/Connectors & References/Phase Splitter
  Phase Splitter1 : ee_lib/Connectors & References/Phase Splitter
  Simulink-PS Converter : nesl_utility/Simulink-PS Converter  PhysicalDomain=network_engine_domain  SubClassName=ps_input  LeftPortType=input  RightPortType=output  PseudoPeriodic=off  Frequencies=[]  NoiseDistribution=none  NoiseParameters=[]  Unit=1  AffineConversion=off  FilteringAndDerivatives=provide  SimscapeFilterOrder=1  InputFilterTimeConstant=0.001  UdotUserProvided=0
  Variable Resistor : fl_lib/Electrical/Electrical Elements/Variable Resistor  Rmin=1e-3 Ohm  thermalEnable=false  thermal_mass=1 J/K  i_specify=off  i_priority=None  i=0 A  i_nominal_specify=off  i_nominal_value=1  i_nominal_unit=A  v_specify=off  v_priority=None  v=0 V  v_nominal_specify=off  v_nominal_value=1  v_nominal_unit=V  T_specify=off  T_priority=None  T=300 K  T_nominal_specify=off  T_nominal_value=1  T_nominal_unit=K
  Variable Resistor1 : fl_lib/Electrical/Electrical Elements/Variable Resistor  Rmin=1e-3 Ohm  thermalEnable=false  thermal_mass=1 J/K  i_specify=off  i_priority=None  i=0 A  i_nominal_specify=off  i_nominal_value=1  i_nominal_unit=A  v_specify=off  v_priority=None  v=0 V  v_nominal_specify=off  v_nominal_value=1  v_nominal_unit=V  T_specify=off  T_priority=None  T=300 K  T_nominal_specify=off  T_nominal_value=1  T_nominal_unit=K
  Variable Resistor2 : fl_lib/Electrical/Electrical Elements/Variable Resistor  Rmin=1e-3 Ohm  thermalEnable=false  thermal_mass=1 J/K  i_specify=off  i_priority=None  i=0 A  i_nominal_specify=off  i_nominal_value=1  i_nominal_unit=A  v_specify=off  v_priority=None  v=0 V  v_nominal_specify=off  v_nominal_value=1  v_nominal_unit=V  T_specify=off  T_priority=None  T=300 K  T_nominal_specify=off  T_nominal_value=1  T_nominal_unit=K
  In : PMIOPort  Side=Left
  ~ : PMIOPort  Port=2  Side=Right
  wires:
  Data Type Conversion/1 -> Open Resistance/1
  BRK/1 -> Data Type Conversion/1
  Open Resistance/1 -> Simulink-PS Converter/1
  connections:
  Phase Splitter1/RConn2 -- Variable Resistor1/RConn1
  Variable Resistor1/LConn2 -- Phase Splitter/RConn2
  Phase Splitter1/RConn3 -- Variable Resistor2/RConn1
  Phase Splitter/RConn1 -- Variable Resistor/LConn2
  Variable Resistor2/LConn2 -- Phase Splitter/RConn3
  Phase Splitter1/RConn1 -- Variable Resistor/RConn1
  Phase Splitter1/LConn1 -- ~/RConn1
  Variable Resistor/LConn1 -- Simulink-PS Converter/RConn1 -- Variable Resistor2/LConn1 -- Variable Resistor1/LConn1
  Phase Splitter/LConn1 -- In/RConn1
